simulink model "Dynamic_Saturation"  (R2025a)
settings: Solver=VariableStepAuto  StartTime=0.0  StopTime=10.0  RelTol=1e-3
settings Model: Creator=xing2  LastModifiedBy=xing2

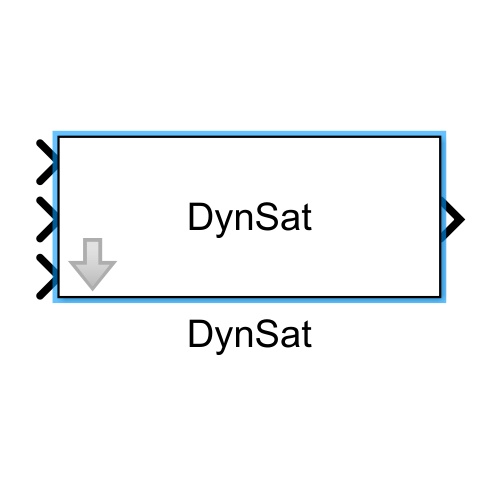
[thumbnail: Simulink's stored preview of the top-level diagram]
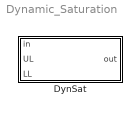
== system Dynamic_Saturation ==
  DynSat : Subsystem
      mask help: Dynamic Saturation with variable limits via input ports
      mask Display: disp('DynSat');

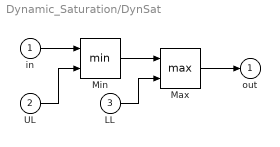
== system Dynamic_Saturation/DynSat ==
  in : Inport
  UL : Inport  Port=2
  LL : Inport  Port=3
  Max : MinMax  Function=max  Inputs=2
  Min : MinMax  Inputs=2
  out : Outport
  wires:
  in/1 -> Min/1
  Max/1 -> out/1
  LL/1 -> Max/2
  UL/1 -> Min/2
  Min/1 -> Max/1
